simulink model "eq_espaco_estados"  (R2021a)
settings: Solver=VariableStepAuto  StartTime=0.0  StopTime=10.0  RelTol=1e-3
values from neighbouring files (symbols this model uses):
  f = 10    [parametros_2a_ordem.m]
  J = 10    [parametros_2a_ordem.m]
  Ka = 10    [parametros_2a_ordem.m]
  Kg = 10    [parametros_2a_ordem.m]
  La = 10    [parametros_2a_ordem.m]
  Ra = 10    [parametros_2a_ordem.m]
undefined symbols (not defined in the file or in its folder): j
settings Model: Creator=Usuário  LastModifiedBy=Usuário

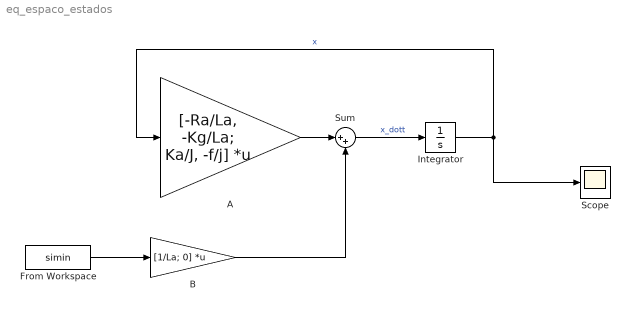
== system eq_espaco_estados ==
  A : Gain  Gain=[-Ra/La, -Kg/La; Ka/J, -f/j]  Multiplication=Matrix(K*u)
  B : Gain  Gain=[1/La; 0]  Multiplication=Matrix(K*u)
  From Workspace : FromWorkspace  VariableName=simin
  Integrator : Integrator
  Scope : Scope
  Sum : Sum  Inputs=|++
  wires:
  B/1 -> Sum/2
  A/1 -> Sum/1
  Sum/1 -> Integrator/1  "x_dott"
  Integrator/1 -> Scope/1, A/1  "x"
  From Workspace/1 -> B/1
